simulink model "TAULab4"  (R2014b)
settings: Solver=ode45  StartTime=0.0  StopTime=10.0  RelTol=1e-3
settings Model: Creator=kiril_000  LastModifiedBy=kiril_000

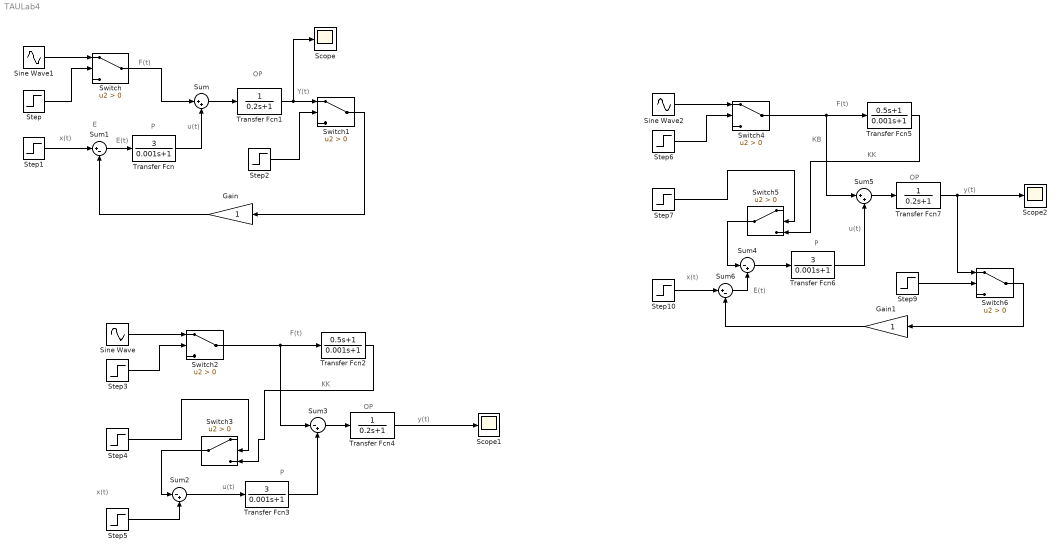
== system TAULab4 ==
  note: Е(t)
  note: КВ
  note: Y(t)
  note: u(t)
  note: F(t)
  note: OP
  note: P
  note: E(t)
  note: Е
  note: x(t)
  note: KK
  note: OP
  note: P
  note: u(t)
  note: F(t)
  note: y(t)
  note: x(t)
  note: KK
  note: OP
  note: P
  note: u(t)
  note: F(t)
  note: y(t)
  note: x(t)
  Gain : Gain
  Gain1 : Gain
  Scope : Scope
      settings: TimeRange=10  YMin=0  YMax=3.5
  Scope1 : Scope
      settings: YMin=-1  YMax=1
  Scope2 : Scope
      settings: YMin=-1  YMax=1  SaveName=ScopeData2
  Sine Wave : Sin  Frequency=10  SampleTime=0
  Sine Wave1 : Sin  Frequency=10  SampleTime=0
  Sine Wave2 : Sin  Frequency=10  SampleTime=0
  Step : Step  SampleTime=2
  Step1 : Step  SampleTime=0
  Step10 : Step  SampleTime=0
  Step2 : Step  SampleTime=6
  Step3 : Step  SampleTime=2
  Step4 : Step  SampleTime=4
  Step5 : Step  SampleTime=0
  Step6 : Step  SampleTime=2
  Step7 : Step  SampleTime=4
  Step9 : Step  SampleTime=6
  Sum : Sum  Inputs=|++
  Sum1 : Sum  Inputs=|+-
  Sum2 : Sum  Inputs=|-+
  Sum3 : Sum  Inputs=|-+
  Sum4 : Sum  Inputs=|-+
  Sum5 : Sum  Inputs=|++
  Sum6 : Sum  Inputs=|+-
  Switch{,1..6} (7 alike) : Switch  Criteria=u2 > Threshold
  Transfer Fcn : TransferFcn  Numerator=[3]  Denominator=[0.001 1]
  Transfer Fcn1 : TransferFcn  Denominator=[0.2 1]
  Transfer Fcn2 : TransferFcn  Numerator=[0.5 1]  Denominator=[0.001 1]
  Transfer Fcn3 : TransferFcn  Numerator=[3]  Denominator=[0.001 1]
  Transfer Fcn4 : TransferFcn  Denominator=[0.2 1]
  Transfer Fcn5 : TransferFcn  Numerator=[0.5 1]  Denominator=[0.001 1]
  Transfer Fcn6 : TransferFcn  Numerator=[3]  Denominator=[0.001 1]
  Transfer Fcn7 : TransferFcn  Denominator=[0.2 1]
  wires:
  Sine Wave1/1 -> Switch/1
  Step/1 -> Switch/2
  Switch/1 -> Sum/1
  Transfer Fcn/1 -> Sum/2
  Sum/1 -> Transfer Fcn1/1
  Step2/1 -> Switch1/2
  Switch1/1 -> Gain/1
  Gain/1 -> Sum1/2
  Sum1/1 -> Transfer Fcn/1
  Step1/1 -> Sum1/1
  Transfer Fcn1/1 -> Switch1/1, Scope/1
  Sine Wave/1 -> Switch2/1
  Step3/1 -> Switch2/2
  Switch2/1 -> Sum3/1, Transfer Fcn2/1
  Transfer Fcn2/1 -> Switch3/3
  Step4/1 -> Switch3/2
  Step5/1 -> Sum2/2
  Sum2/1 -> Transfer Fcn3/1
  Transfer Fcn3/1 -> Sum3/2
  Sum3/1 -> Transfer Fcn4/1
  Transfer Fcn4/1 -> Scope1/1
  Sine Wave2/1 -> Switch4/1
  Step6/1 -> Switch4/2
  Switch4/1 -> Sum5/1, Transfer Fcn5/1
  Transfer Fcn5/1 -> Switch5/3
  Step7/1 -> Switch5/2
  Switch5/1 -> Sum4/1
  Sum4/1 -> Transfer Fcn6/1
  Transfer Fcn6/1 -> Sum5/2
  Sum5/1 -> Transfer Fcn7/1
  Transfer Fcn7/1 -> Scope2/1, Switch6/1
  Switch6/1 -> Gain1/1
  Gain1/1 -> Sum6/2
  Step9/1 -> Switch6/2
  Step10/1 -> Sum6/1
  Sum6/1 -> Sum4/2
  Switch3/1 -> Sum2/1
